simulink model "RainSnsrWiperMot"  (R2020b)
settings: Solver=FixedStepDiscrete  StartTime=0.0  StopTime=20  FixedStep=0.01  RelTol=1e-3
undefined symbols (not defined in the file): sigbuilder_block
libraries: simulink x1
settings Model: Creator=Emiliano  LastModifiedBy=Emiliano
settings OptimizationCC: DefaultParameterBehavior=Inlined  UseDivisionForNetSlopeComputation=on  GainParamInheritBuiltInType=on  UseFloatMulNetSlope=on  InlineInvariantSignals=on  PassReuseOutputArgsAs=Individual arguments  ZeroExternalMemoryAtStartup=off  ZeroInternalMemoryAtStartup=off  NoFixptDivByZeroProtection=on  EfficientFloat2IntCast=on  LifeSpan=1  OptimizeBlockOrder=speed  DifferentSizesBufferReuse=on  EfficientTunableParamExpr=on
settings DebuggingCC: ParameterTunabilityLossMsg=error
settings HardwareCC: ProdLongLongMode=on
settings SFSimCC: MATLABDynamicMemAlloc=off
settings RTWCC: Description=Embedded Coder  SystemTargetFile=ert.tlc  TemplateMakefile=ert_default_tmf
settings CodeAppCC: ForceParamTrailComments=on  IgnoreCustomStorageClasses=off  OperatorAnnotations=on  SimulinkDataObjDesc=on  SFDataObjDesc=on  CustomSymbolStrGlobalVar=rt$N$M  CustomSymbolStrType=$N$M  CustomSymbolStrFcn=$N$M$F  CustomSymbolStrMacro=$N$M  InsertBlockDesc=on
settings ERTTargetCC: TargetLangStandard=C99 (ISO)  GenerateSampleERTMain=on  IncludeMdlTerminateFcn=off  CombineSignalStateStructs=on  SupportComplex=off  SupportNonInlinedSFcns=on  InlinedParameterPlacement=NonHierarchical  ERTCustomFileTemplate=example_file_process.tlc  ERTFilePackagingFormat=CompactWithDataFile

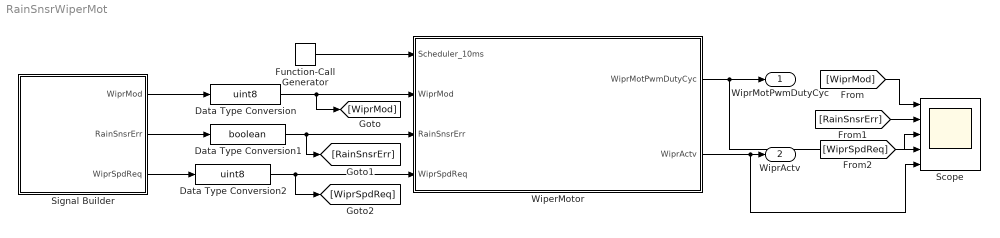
== system RainSnsrWiperMot ==
  Data Type Conversion : DataTypeConversion  OutDataTypeStr=uint8
  Data Type Conversion1 : DataTypeConversion  OutDataTypeStr=boolean
  Data Type Conversion2 : DataTypeConversion  OutDataTypeStr=uint8
  Function-Call Generator : simulink/Ports & Subsystems/Function-Call Generator  sample_time=10e-3  numberOfIterations=1  DisallowWideOutput=off
  Scope : Scope  NumInputPorts=5
  Signal Builder : Subsystem  Tag=STV Subsys  LoadFcn=sigbuilder_block('load');  StartFcn=sigbuilder_block('start');  StopFcn=sigbuilder_block('stop');  ClipboardFcn=sigbuilder_block('clipboard');  mask(Sigbuilder block){tuvar=[0:10]}
      mask help: Simulink:masks:SigbuilderBlock_MD
      mask init:
      | if ~strcmp(get_param(bdroot(gcbh),'SimulationStatus'),'stopped') tuvar = sigbuilder_block('maskInit'); end
      settings: CopyFcn=sigbuilder_block('copy');  DeleteFcn=sigbuilder_block('delete');  ModelCloseFcn=sigbuilder_block('modelClose');  PreSaveFcn=sigbuilder_block('preSave');  PauseFcn=sigbuilder_block('pause');  ContinueFcn=sigbuilder_block('continue');  NameChangeFcn=sigbuilder_block('namechange');  OpenFcn=sigbuilder_block('open',[6 30 1188 546.75 ]);  CloseFcn=sigbuilder_block('close');
      mask Display: plot(0, 0, 100, 100,[2, 2, 32, 32, 2], [68, 8, 8, 68, 68],[32, 2], [38, 38], [32, 19, 2],[53, 60, 44], [32, 17, 17, 2],[16, 16, 31, 31]);txt = getActiveGroup(gcbh);text(2, 100, txt,'verticalAlignment', 'top');
  WiperMotor : Subsystem
  WiprMotPwmDutyCyc : Outport
  WiprActv : Outport  Port=2
  wires:
  Function-Call Generator/1 -> WiperMotor/1(Scheduler_10ms)
  WiperMotor/1(WiprMotPwmDutyCyc) -> WiprMotPwmDutyCyc/1, Scope/4
  WiperMotor/2(WiprActv) -> Scope/5, WiprActv/1
  Signal Builder/2(RainSnsrErr) -> Data Type Conversion1/1
  Signal Builder/1(WiprMod) -> Data Type Conversion/1
  Signal Builder/3(WiprSpdReq) -> Data Type Conversion2/1
  [WiprMod] -> Scope/1
  [RainSnsrErr] -> Scope/2
  [WiprSpdReq] -> Scope/3
  Data Type Conversion/1 -> WiperMotor/2(WiprMod), [WiprMod]
  Data Type Conversion1/1 -> WiperMotor/3(RainSnsrErr), [RainSnsrErr]
  Data Type Conversion2/1 -> [WiprSpdReq], WiperMotor/4(WiprSpdReq)

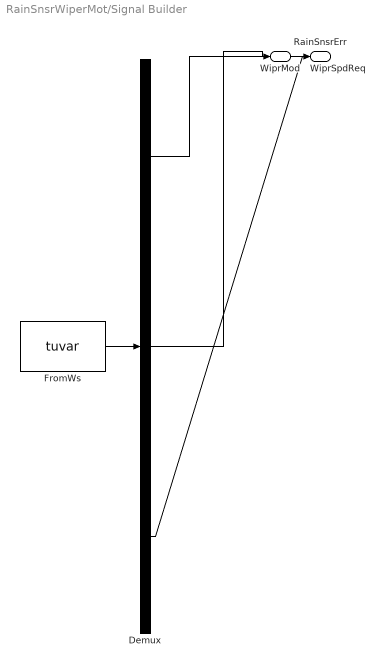
== system RainSnsrWiperMot/Signal Builder ==
  Demux : Demux  Tag=STV Demux  Outputs=3
      settings: DisplayOption=none
  FromWs : FromWorkspace  Tag=STV FromWs  VariableName=tuvar
      SigBuilderData=|
      | common.afterFinalStr = 'Extrapolate'
      | common.sampleTime = 0
      | dataSet.timeRange = [0 20]
      | dataSet.name = 'Group 1'
      | sbobj.Groups.Name = 'Group 1'
      | sbobj.Groups.Signals(1).Name = 'WiprMod'
      | sbobj.Groups.Signals(1).XData = [0 1 2 3 4 5 6 20]
      | sbobj.Groups.Signals(1).YData = [0 0 2 2 3 3 1 1]
      | sbobj.Groups.Signals(2).Name = 'RainSnsrErr'
      | sbobj.Groups.Signals(2).XData = [0 14 15 16 20]
      | sbobj.Groups.Signals(2).YData = [0 0 1 0 0]
      | sbobj.Groups.Signals(3).Name = 'WiprSpdReq'
      | sbobj.Groups.Signals(3).XData = [0 7 14 20]
      | sbobj.Groups.Signals(3).YData = [0 0 6 6]
      | sbobj.Groups.TimeRange = [0 20]
  WiprMod : Outport  Tag=STV Outport
  RainSnsrErr : Outport  Tag=STV Outport  Port=2
  WiprSpdReq : Outport  Tag=STV Outport  Port=3
  wires:
  Demux/1 -> WiprMod/1
  FromWs/1 -> Demux/1
  Demux/2 -> RainSnsrErr/1
  Demux/3 -> WiprSpdReq/1

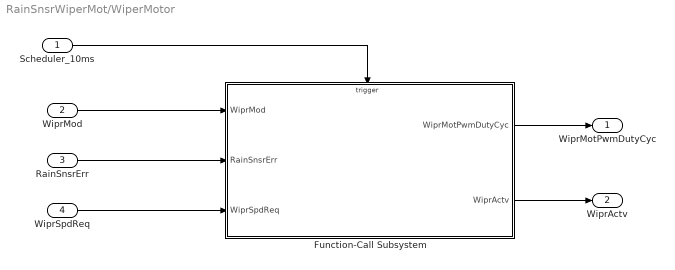
== system RainSnsrWiperMot/WiperMotor ==
  Scheduler_10ms : Inport
  WiprMod : Inport  Port=2  OutDataTypeStr=uint8
  RainSnsrErr : Inport  Port=3  OutDataTypeStr=boolean
  WiprSpdReq : Inport  Port=4  OutDataTypeStr=uint8
  Function-Call Subsystem : Subsystem  TreatAsAtomicUnit=on
  WiprMotPwmDutyCyc : Outport
  WiprActv : Outport  Port=2
  wires:
  Function-Call Subsystem/1(WiprMotPwmDutyCyc) -> WiprMotPwmDutyCyc/1
  WiprSpdReq/1 -> Function-Call Subsystem/3(WiprSpdReq)
  Scheduler_10ms/1 -> Function-Call Subsystem/Trigger
  Function-Call Subsystem/2(WiprActv) -> WiprActv/1
  RainSnsrErr/1 -> Function-Call Subsystem/2(RainSnsrErr)
  WiprMod/1 -> Function-Call Subsystem/1(WiprMod)

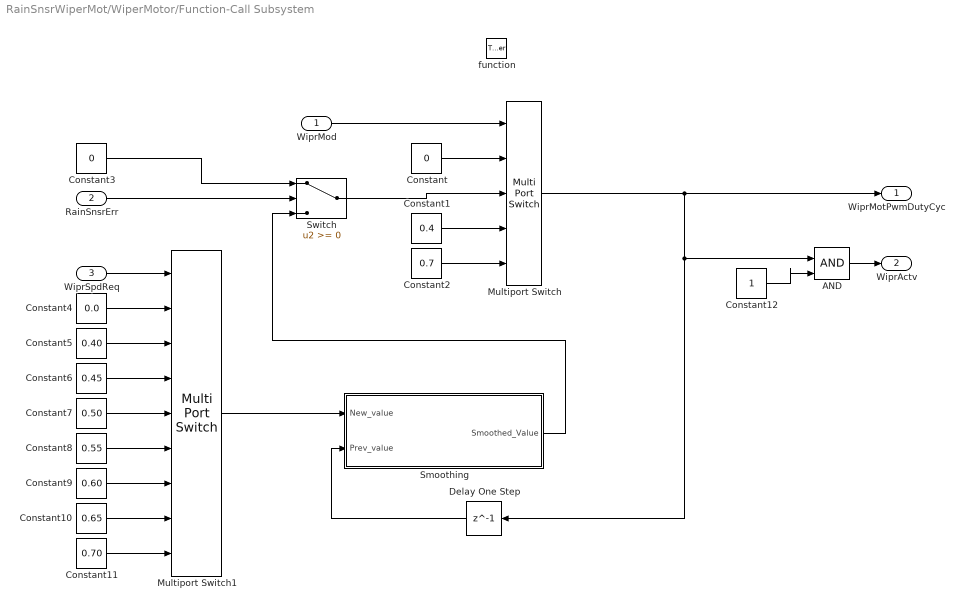
== system RainSnsrWiperMot/WiperMotor/Function-Call Subsystem ==
  WiprMod : Inport  OutDataTypeStr=uint8
  RainSnsrErr : Inport  Port=2  OutDataTypeStr=boolean
  WiprSpdReq : Inport  Port=3  OutDataTypeStr=uint8
  function : TriggerPort  TriggerType=function-call  VariantControl=Variant
  AND : Logic  IconShape=distinctive  AllPortsSameDT=off  OutDataTypeStr=boolean
  Constant : Constant  Value=0
  Constant1 : Constant  Value=0.4
  Constant10 : Constant  Value=0.65
  Constant11 : Constant  Value=0.70
  Constant12 : Constant
  Constant2 : Constant  Value=0.7
  Constant3 : Constant  Value=0
  Constant4 : Constant  Value=0.0
  Constant5 : Constant  Value=0.40
  Constant6 : Constant  Value=0.45
  Constant7 : Constant  Value=0.50
  Constant8 : Constant  Value=0.55
  Constant9 : Constant  Value=0.60
  Delay One Step : Delay  DelayLength=1
  Multiport Switch : MultiPortSwitch  DataPortOrder=Zero-based contiguous  Inputs=4  zeroidx=on
  Multiport Switch1 : MultiPortSwitch  DataPortOrder=Zero-based contiguous  Inputs=8  zeroidx=on
  Smoothing : Subsystem
  Switch : Switch  OutDataTypeStr=boolean  InputSameDT=on
  WiprMotPwmDutyCyc : Outport  OutDataTypeStr=double
  WiprActv : Outport  Port=2  OutDataTypeStr=boolean
  wires:
  WiprMod/1 -> Multiport Switch/1
  Constant/1 -> Multiport Switch/2
  Constant2/1 -> Multiport Switch/5
  Constant1/1 -> Multiport Switch/4
  RainSnsrErr/1 -> Switch/2
  Constant3/1 -> Switch/1
  Switch/1 -> Multiport Switch/3
  WiprSpdReq/1 -> Multiport Switch1/1
  Constant4/1 -> Multiport Switch1/2
  Constant5/1 -> Multiport Switch1/3
  Constant6/1 -> Multiport Switch1/4
  Constant7/1 -> Multiport Switch1/5
  Constant8/1 -> Multiport Switch1/6
  Constant9/1 -> Multiport Switch1/7
  Constant10/1 -> Multiport Switch1/8
  Constant11/1 -> Multiport Switch1/9
  AND/1 -> WiprActv/1
  Multiport Switch/1 -> WiprMotPwmDutyCyc/1, AND/1, Delay One Step/1
  Constant12/1 -> AND/2
  Multiport Switch1/1 -> Smoothing/1(New_value)
  Delay One Step/1 -> Smoothing/2(Prev_value)
  Smoothing/1(Smoothed_Value) -> Switch/3

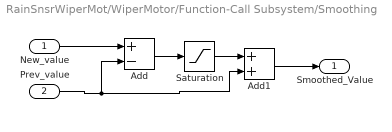
== system RainSnsrWiperMot/WiperMotor/Function-Call Subsystem/Smoothing ==
  New_value : Inport
  Prev_value : Inport  Port=2
  Add : Sum  Inputs=+-
  Add1 : Sum
  Saturation : Saturate  UpperLimit=0.005  LowerLimit=-0.005
  Smoothed_Value : Outport
  wires:
  Prev_value/1 -> Add/2, Add1/2
  New_value/1 -> Add/1
  Saturation/1 -> Add1/1
  Add1/1 -> Smoothed_Value/1
  Add/1 -> Saturation/1
